simulink model "ex2"  (R2015a)
settings: Solver=ode4  StartTime=0.0  StopTime=20.0  FixedStep=0.01  RelTol=1e-3
values from neighbouring files (symbols this model uses):
  A = [0 0 0; 1 0 -1; 0 1 2]    [ex1.m]
  B = [0 -1; 1 0; 0 1]    [ex1.m]
  C = [1 0 1]    [ex1.m]
settings Model: Creator=Cazan Bogdan  LastModifiedBy=andre

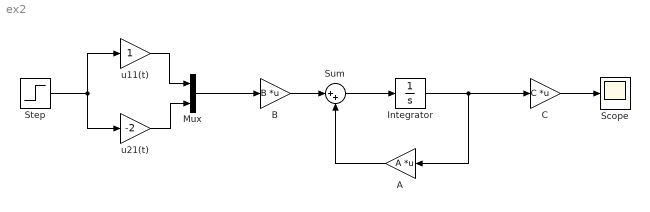
== system ex2 ==
  A : Gain  Gain=A  Multiplication=Matrix(K*u)
  B : Gain  Gain=B  Multiplication=Matrix(K*u)
  C : Gain  Gain=C  Multiplication=Matrix(K*u)
  Integrator : Integrator
  Mux : Mux  Inputs=2
  Scope : Scope
      settings: TimeRange=20  YMin=-5000000000  YMax=3000000000
  Step : Step  SampleTime=0
  Sum : Sum  Inputs=|++
  u11(t) : Gain
  u21(t) : Gain  Gain=-2
  wires:
  Step/1 -> u21(t)/1, u11(t)/1
  u11(t)/1 -> Mux/1
  u21(t)/1 -> Mux/2
  Mux/1 -> B/1
  B/1 -> Sum/1
  Sum/1 -> Integrator/1
  Integrator/1 -> A/1, C/1
  A/1 -> Sum/2
  C/1 -> Scope/1
